simulink model "Phase_Recovery_Data_Aided"  (Simulink 8.6)
settings: Solver=FixedStepDiscrete  StartTime=0  StopTime=inf  RelTol=1e-3
InitFcn:
  | % Trainingssequenz
  | trainseq=1/sqrt(2) * ((2*randi([0 1],32,1)-1) + 1i * (2*randi([0 1],32,1)-1));
libraries: commdigbbndpm3 x2, commchan3 x1, dspsrcs4 x1, commsink2 x1, simulink x1, commrandsrc2 x1
settings Model: Creator=schwall  LastModifiedBy=wunsch
settings DataIOCC: SaveOutput=off  SignalLogging=off  SaveTime=off
settings DebuggingCC: InheritedTsInSrcMsg=none  FcnCallInpInsideContextMsg=UseLocalSettings
settings SFSimCC: SimParseCustomCode=off
settings ConfigComp: CovSFcnEnable=off

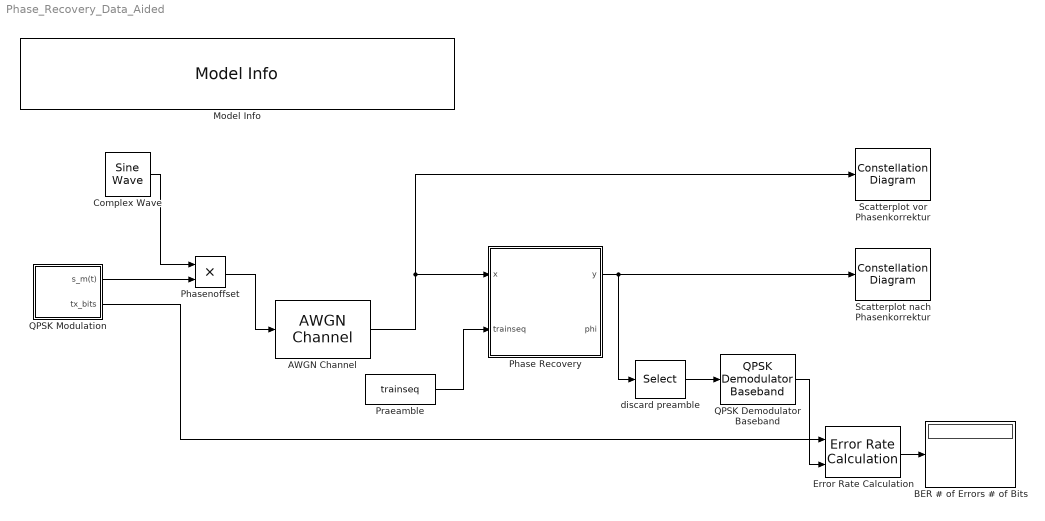
== system Phase_Recovery_Data_Aided ==
  AWGN Channel : commchan3/AWGN Channel  InputProcessing=Columns as channels (frame based)  seed=67  noiseMode="Signal to noise ratio  (Eb/No)"  EbNodB=25  EsNodB=10  SNRdB=10  bitsPerSym=1  Ps=1  Tsym=0.128/160  variance=1
  BER # of Errors # of Bits : Display
  Complex Wave : dspsrcs4/Sine Wave  Amplitude=1  Frequency=0  Phase=0  SampleMode=Discrete  OutComplex=Complex  CompMethod=Trigonometric fcn  TableSize=Speed  SampleTime=0.128/160  SamplesPerFrame=160  ResetState=Restart at time zero  OutputFrames=on  dataType=double  wordLen=16  udDataType=sfix(16)  fracBitsMode=Best precision  numFracBits=15  OutDataTypeStr=double  LastOutDataTypeStr=double
  Error Rate Calculation : commsink2/Error Rate Calculation  N=0  st_delay=0  cp_mode=Entire frame  subframe=[]  PMode=Port  WsName=ErrorVec  RsMode2=off  stop=off  numErr=100  maxBits=1e6
  Model Info : simulink/Model-Wide Utilities/Model Info  BlockCM=None  Frame=on  DisplayStringWithTags=|  HorizontalTextAlignment=Left  LeftAlignmentValue=0.02  SourceBlockDiagram=Phase_Recovery_Data_Aided  TagMaxNumber=20
      | Demo Phase Recovery (Open Loop)
      | Vorlesung Nachrichtentechnik II
      | Institut fuer Nachrichtentechnik (CEL)
  Phase Recovery : MATLAB Function  TreatAsAtomicUnit=on
  Phasenoffset : Product  RndMeth=Zero
  Praeamble : Constant  Value=trainseq  VectorParams1D=off  FramePeriod=-1
      settings: SamplingMode=Frame based
  QPSK Demodulator Baseband : commdigbbndpm3/QPSK Demodulator Baseband  Ph=pi/4  Dec=Gray  OutType=Bit  DecType=Hard decision  VarSource=Dialog  Variance=1  outDtype1=Inherit via internal rule  outDtype2=Inherit via internal rule  derotateFactorWordLen=16
  QPSK Modulation : Subsystem
  Scatterplot nach Phasenkorrektur : ConstellationDiagram  Tag=ScatterPlot
  Scatterplot vor Phasenkorrektur : ConstellationDiagram  Tag=ScatterPlot
  discard preamble : Selector  NumberOfDimensions=2  InputPortWidth=3  IndexOptions=Index vector (dialog),Select all  Indices=[33:160],1  OutputSizes=1,1
  wires:
  QPSK Modulation/1(s_m(t)) -> Phasenoffset/2
  Praeamble/1 -> Phase Recovery/2(trainseq)
  Phase Recovery/1(y) -> Scatterplot nach Phasenkorrektur/1, discard preamble/1
  discard preamble/1 -> QPSK Demodulator Baseband/1
  AWGN Channel/1 -> Phase Recovery/1(x), Scatterplot vor Phasenkorrektur/1
  Phasenoffset/1 -> AWGN Channel/1
  Complex Wave/1 -> Phasenoffset/1
  QPSK Demodulator Baseband/1 -> Error Rate Calculation/2
  QPSK Modulation/2(tx_bits) -> Error Rate Calculation/1
  Error Rate Calculation/1 -> BER # of Errors # of Bits/1

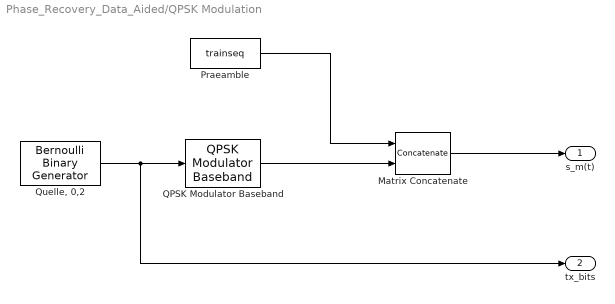
== system Phase_Recovery_Data_Aided/QPSK Modulation ==
  Matrix Concatenate : Concatenate  Mode=Multidimensional array
  Praeamble : Constant  Value=trainseq  VectorParams1D=off  FramePeriod=-1
      settings: SamplingMode=Frame based
  QPSK Modulator Baseband : commdigbbndpm3/QPSK Modulator Baseband  InType=Bit  Enc=Gray  Ph=pi/4  outDtype=double  outWordLen=16  outUDDataType=sfix(16)  outFracLenMode=Best precision  outFracLen=15
  "Quelle, 0,2" : commrandsrc2/Bernoulli Binary Generator  P=0.5  seed=61  Ts=1/1000/2  frameBased=on  sampPerFrame=256  orient=off  outDataType=double
  s_m(t) : Outport
  tx_bits : Outport  Port=2
  wires:
  "Quelle, 0,2"/1 -> QPSK Modulator Baseband/1, tx_bits/1
  QPSK Modulator Baseband/1 -> Matrix Concatenate/2
  Praeamble/1 -> Matrix Concatenate/1
  Matrix Concatenate/1 -> s_m(t)/1

== matlab function Phase Recovery ==
  data: x input double; y output double; trainseq input double; phi output double
function [y,phi] = recovery(x,trainseq)
%#codegen

%%%%%%%%%%%%%%%%%%%%%%%%%%%%%%%%%%%%%%%%%%%%%%%%%%%%%%%%%%%%%%%%%%%%%%%%%%%
% Initalisierung
%%%%%%%%%%%%%%%%%%%%%%%%%%%%%%%%%%%%%%%%%%%%%%%%%%%%%%%%%%%%%%%%%%%%%%%%%%%

L0       = 32;                      % Beobachtungsdauer


%%%%%%%%%%%%%%%%%%%%%%%%%%%%%%%%%%%%%%%%%%%%%%%%%%%%%%%%%%%%%%%%%%%%%%%%%%%
% Phase Recovery (Open Loop)
%%%%%%%%%%%%%%%%%%%%%%%%%%%%%%%%%%%%%%%%%%%%%%%%%%%%%%%%%%%%%%%%%%%%%%%%%%%

% Bestimmung des Phasenoffsets
phi = angle( sum( conj(trainseq).* x(1:L0,1) ) );

% Korrektur des Empfangssignals
y = x * exp(1i * (-phi));
